simulink model "EX6_1C2_Buck_Converter_CCM_Design"  (R2024a)
settings: Solver=VariableStepAuto  StartTime=0.0  StopTime=0.0005  RelTol=1e-3
libraries: spsGroundLib x4, spsSeriesRLCBranchLib x3, spsCurrentMeasurementLib x3, eeRmsMeasurement x2, spsVoltageMeasurementLib x2, spsDCVoltageSourceLib x1, spsDiodeLib x1, spsIdealSwitchLib x1, spspowerguiLib x1
settings Model: Creator=mca04  LastModifiedBy=mca04

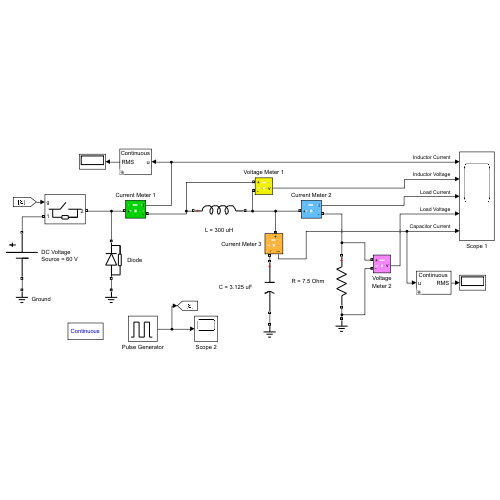
[thumbnail: Simulink's stored preview of the top-level diagram]
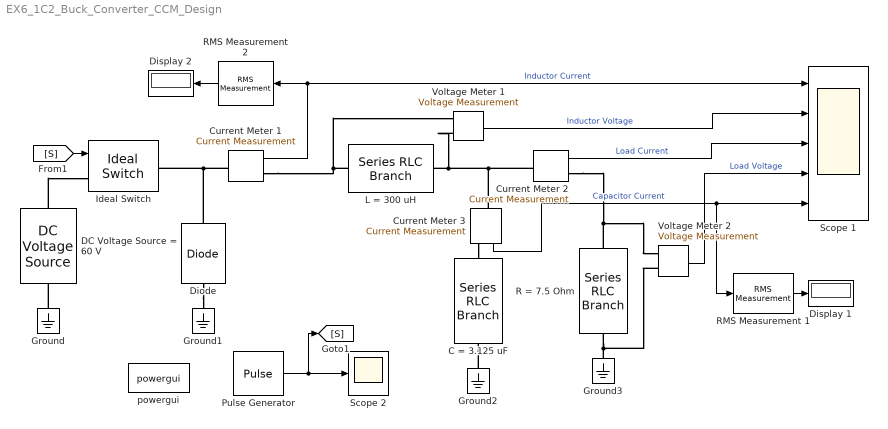
== system EX6_1C2_Buck_Converter_CCM_Design ==
  C = 3.125 uF : spsSeriesRLCBranchLib/Series RLC Branch  LConnTagsString=__new0  RConnTagsString=__new0  BranchType=C  Resistance=1  Inductance=150e-6  SetiL0=off  InitialCurrent=0  Capacitance=3.125e-6  Setx0=off  InitialVoltage=0  Measurements=None
  Current Meter 1 : spsCurrentMeasurementLib/Current Measurement  PhasorSimulation=off  OutputType=Complex  PSBequivalent=0
  Current Meter 2 : spsCurrentMeasurementLib/Current Measurement  PhasorSimulation=off  OutputType=Complex  PSBequivalent=0
  Current Meter 3 : spsCurrentMeasurementLib/Current Measurement  PhasorSimulation=off  OutputType=Complex  PSBequivalent=0
  DC Voltage Source = 60 V : spsDCVoltageSourceLib/DC Voltage Source  Amplitude=60  Measurements=Voltage
  Diode : spsDiodeLib/Diode  Ron=0.001  Lon=0  Vf=0.001  IC=0  UseSnubber=0  Rs=1e12  Cs=1e-12  Measurements=off
  Display 1 : Display
  Display 2 : Display
  Ground{,1..3} (4 alike) : spsGroundLib/Ground  LConnTagsString=a
  Ideal Switch : spsIdealSwitchLib/Ideal Switch  Ron=0.001  Lon=0  IC=0  Rs=1e12  Cs=inf  Measurements=off
  L = 300 uH : spsSeriesRLCBranchLib/Series RLC Branch  LConnTagsString=__new0  RConnTagsString=__new0  BranchType=L  Resistance=1  Inductance=300e-6  SetiL0=off  InitialCurrent=0  Capacitance=1e-6  Setx0=off  InitialVoltage=0  Measurements=None
  Pulse Generator : DiscretePulseGenerator  PulseType=Time based  Period=1/1e5  PulseWidth=25
  R = 7.5 Ohm : spsSeriesRLCBranchLib/Series RLC Branch  LConnTagsString=__new0  RConnTagsString=__new0  BranchType=R  Resistance=7.5  Inductance=150e-6  SetiL0=off  InitialCurrent=0  Capacitance=100e-6  Setx0=off  InitialVoltage=0  Measurements=None
  RMS Measurement 1 : eeRmsMeasurement/RMS Measurement  LabelModeActiveChoice=Total  F=1e5  SpecifyHarmonics=off  K=[0 1 2]  Ts=0
      settings: LibrarySourceBlock=|
      | ee_sl_lib/Measurements/RMS
      | Measurement
  RMS Measurement 2 : eeRmsMeasurement/RMS Measurement  LabelModeActiveChoice=Total  F=1e5  SpecifyHarmonics=off  K=[0 1 2]  Ts=0
      settings: LibrarySourceBlock=|
      | ee_sl_lib/Measurements/RMS
      | Measurement
  Scope 1 : Scope  NumInputPorts=5
  Scope 2 : Scope
  Voltage Meter 2 : spsVoltageMeasurementLib/Voltage Measurement  PhasorSimulation=off  OutputType=Complex  PSBequivalent=0
  Voltage Meter 1 : spsVoltageMeasurementLib/Voltage Measurement  PhasorSimulation=off  OutputType=Complex  PSBequivalent=0
  powergui : spspowerguiLib/powergui  Priority=1  SimulationMode=Continuous  SampleTime=50e-6  frequency=60  Iterations=50  frequencyindice=0  Pbase=100e6  ErrMax=1e-4  UnitsV=kV  UnitsW=MW  buscounter=0  FunctionMessages=off  echomessages=off  EnableUseOfTLC=off  CurrentSourceSwitches=off  DisableSnubberDevices=off  DisableRonSwitches=off  DisableVfSwitches=off  DisplayEquations=off  AutomaticDiscreteSolvers=off  SolverType=Tustin/Backward Euler (TBE)  Interpol=off  ExternalGateDelay=off  methode=off  Ts=100  x0status=blocks  SPID=on  SwTol=0  HookPort=off  NonlinearTolerance=1e-4  nMaxIteration=100  ContinueOnMaxIteration=off  RestoreLinks=warning  ResistiveCurrentMeasurement=off  Frange=[0:2:500]  Ylog=off  Xlog=on  ShowGrid=off  save=off  variable=ZData  structure=0  ZoomFFT=off  StartTime=0.0  cycles=1  DisplayStyle=1  fundamental=60  FreqAxis=off  MaxFrequency=1000  frequencyindicesteady=1  RmsSteady=1  display=off
  wires:
  Pulse Generator/1 -> [S], Scope 2/1
  [S] -> Ideal Switch/1
  Voltage Meter 2/1 -> Scope 1/4  "Load Voltage"
  Voltage Meter 1/1 -> Scope 1/2  "Inductor Voltage"
  Current Meter 2/1 -> Scope 1/3  "Load Current"
  Current Meter 1/1 -> Scope 1/1, RMS Measurement 2/1  "Inductor Current"
  Current Meter 3/1 -> Scope 1/5, RMS Measurement 1/1  "Capacitor Current"
  RMS Measurement 1/1 -> Display 1/1
  RMS Measurement 2/1 -> Display 2/1
  connections:
  DC Voltage Source = 60 V/RConn1 -- Ideal Switch/LConn1
  L = 300 uH/LConn1 -- Current Meter 1/RConn1 -- Voltage Meter 1/LConn1
  R = 7.5 Ohm/LConn1 -- Current Meter 2/RConn1 -- Voltage Meter 2/LConn1
  Ground/LConn1 -- DC Voltage Source = 60 V/LConn1
  Ground2/LConn1 -- C = 3.125 uF/RConn1
  Diode/LConn1 -- Ground1/LConn1
  Current Meter 2/LConn1 -- Current Meter 3/LConn1 -- Voltage Meter 1/LConn2 -- L = 300 uH/RConn1
  Voltage Meter 2/LConn2 -- Ground3/LConn1 -- R = 7.5 Ohm/RConn1
  Diode/RConn1 -- Ideal Switch/RConn1 -- Current Meter 1/LConn1
  Current Meter 3/RConn1 -- C = 3.125 uF/LConn1
